simulink model "ToggleLEDOnRisingEdge"  (R2025a)
settings: Solver=VariableStepAuto  StartTime=0.0  StopTime=10.0  RelTol=1e-3
libraries: simulink x1
settings Model: Creator=mahij  LastModifiedBy=mahij

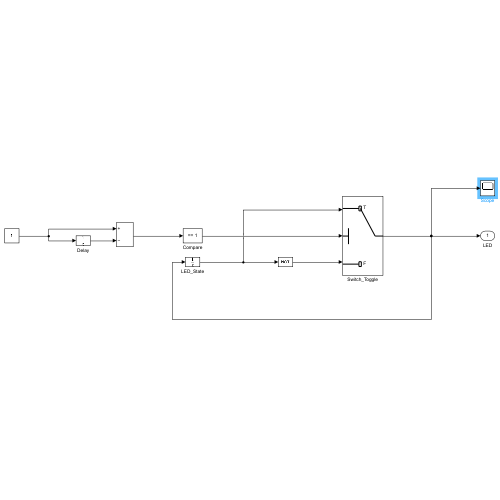
[thumbnail: Simulink's stored preview of the top-level diagram]
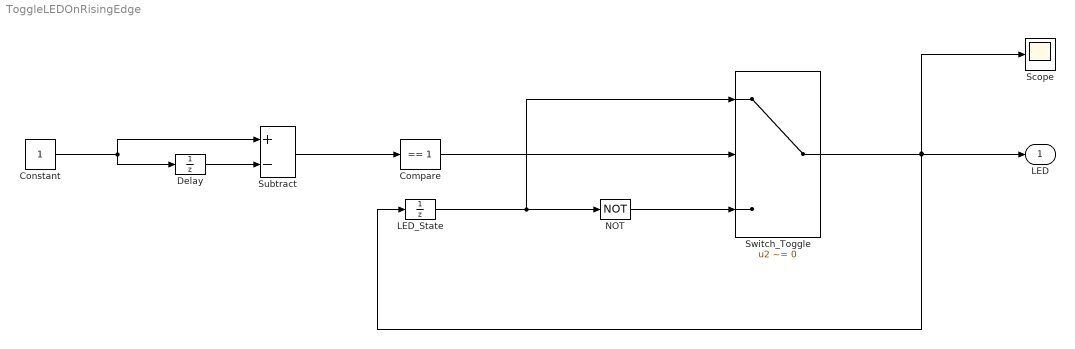
== system ToggleLEDOnRisingEdge ==
  Compare : simulink/Logic and Bit Operations/Compare To Constant  relop===  const=1  OutDataTypeStr=boolean
  Constant : Constant
  Delay : UnitDelay  SampleTime=0.1  HasFrameUpgradeWarning=on
  LED_State : UnitDelay  SampleTime=0.1  HasFrameUpgradeWarning=on
  NOT : Logic  Operator=NOT  AllPortsSameDT=off  OutDataTypeStr=boolean
  Scope : Scope
      settings: ActiveDisplayYMinimum=-0.12499999999999997  ActiveDisplayYMaximum=1.125
  Subtract : Sum  Inputs=+-
  Switch_Toggle : Switch  Criteria=u2 ~= 0  Threshold=0.5  SaturateOnIntegerOverflow=off  InputSameDT=off
  LED : Outport
  wires:
  Constant/1 -> Delay/1, Subtract/1
  Delay/1 -> Subtract/2
  Subtract/1 -> Compare/1
  LED_State/1 -> Switch_Toggle/1, NOT/1
  Compare/1 -> Switch_Toggle/2
  NOT/1 -> Switch_Toggle/3
  Switch_Toggle/1 -> Scope/1, LED/1, LED_State/1
